simulink model "P1_3"  (R2020b)
settings: Solver=VariableStepAuto  StartTime=0.0  StopTime=300  RelTol=1e-3
undefined symbols (not defined in the file): b, Jm, Ke, Kt, La, Ra
libraries: simulink x1
settings Model: Creator=kxt12  LastModifiedBy=kxt12

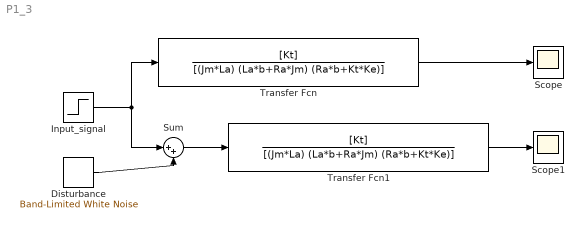
== system P1_3 ==
  Disturbance : simulink/Sources/Band-Limited White Noise  Cov=[0.7]  Ts=0.1  seed=[23341]
  Input_signal : Step  After=20  SampleTime=0
  Scope : Scope
  Scope1 : Scope
  Sum : Sum  Inputs=|++
  Transfer Fcn : TransferFcn  Numerator=[Kt]  Denominator=[(Jm*La) (La*b+Ra*Jm) (Ra*b+Kt*Ke)]
  Transfer Fcn1 : TransferFcn  Numerator=[Kt]  Denominator=[(Jm*La) (La*b+Ra*Jm) (Ra*b+Kt*Ke)]
  wires:
  Input_signal/1 -> Sum/1, Transfer Fcn/1
  Transfer Fcn/1 -> Scope/1
  Transfer Fcn1/1 -> Scope1/1
  Sum/1 -> Transfer Fcn1/1
  Disturbance/1 -> Sum/2
